simulink model "OLvsCL"  (Simulink 8.0)
settings: Solver=ode45  StartTime=0.0  StopTime=10.0  RelTol=1e-3
libraries: NbLibrary x10, cstblocks x7
settings Model: Creator=vaadya  LastModifiedBy=ccw
settings DataIOCC: SignalLoggingSaveFormat=ModelDataLogs
settings OptimizationCC: ExpressionDepthLimit=128
settings DebuggingCC: UnderspecifiedInitializationDetection=Simplified  MergeDetectMultiDrivingBlocksExec=error  SolverPrmCheckMsg=none  FcnCallInpInsideContextMsg=EnableAllAsWarning  FrameProcessingCompatibilityMsg=error  StateNameClashWarn=none
settings CodeAppCC: CustomSymbolStrType=$N$R$M_T
settings GRTTargetCC: CodeReplacementLibrary=C89/C90 (ANSI)  CombineOutputUpdateFcns=off  GRTInterface=on

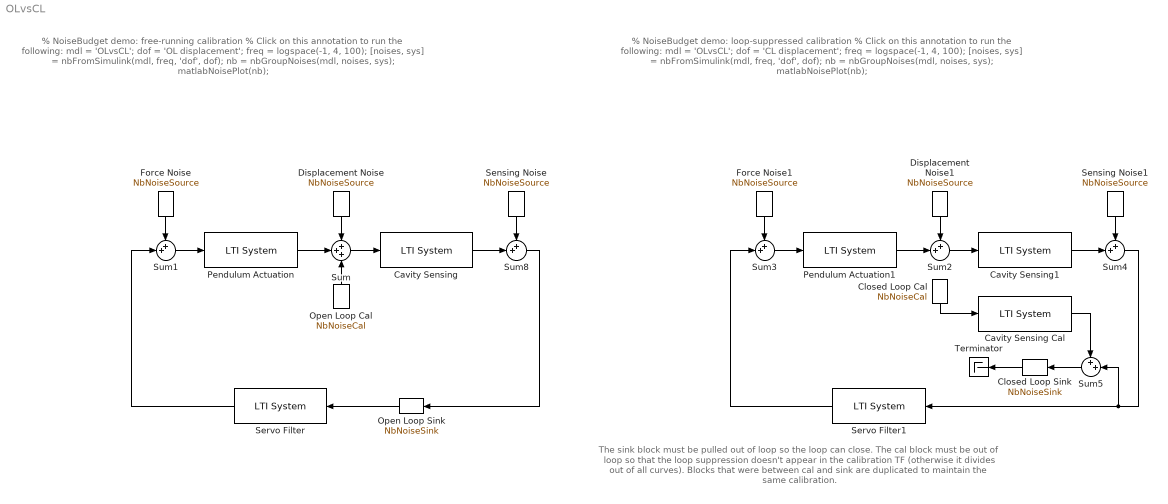
== system OLvsCL ==
  note: The sink block must be pulled out of loop so the loop can close.
      |
      | The cal block must be out of loop so that the loop suppression
      | doesn't appear in the calibration TF (otherwise it divides out of all
      | curves). Blocks that were between cal and sink are duplicated to
      | maintain the same calibration.
  note: % NoiseBudget demo: free-running calibration
      |   % Click on this annotation to run the following:
      |   mdl = 'OLvsCL';
      |   dof = 'OL displacement';
      |   freq = logspace(-1, 4, 100);
      |   [noises, sys] = nbFromSimulink(mdl, freq, 'dof', dof);
      |   nb = nbGroupNoises(mdl, noises, sys);
      |   matlabNoisePlot(nb);
  note: % NoiseBudget demo: loop-suppressed calibration
      |   % Click on this annotation to run the following:
      |   mdl = 'OLvsCL';
      |   dof = 'CL displacement';
      |   freq = logspace(-1, 4, 100);
      |   [noises, sys] = nbFromSimulink(mdl, freq, 'dof', dof);
      |   nb = nbGroupNoises(mdl, noises, sys);
      |   matlabNoisePlot(nb);
  Cavity Sensing : cstblocks/LTI System  sys=zpk([],-2*pi*[1000],2*pi*1000)  IC=[]
  Cavity Sensing Cal : cstblocks/LTI System  sys=zpk([],-2*pi*[1000],2*pi*1000)  IC=[]
  Cavity Sensing1 : cstblocks/LTI System  sys=zpk([],-2*pi*[1000],2*pi*1000)  IC=[]
  Closed Loop Cal : NbLibrary/NbNoiseCal  Tag=NbNoiseCal  dof='CL displacement'  unit='m/rtHz'
      settings: AttributesFormatString=%<Tag>
  Closed Loop Sink : NbLibrary/NbNoiseSink  Tag=NbNoiseSink  dof='CL displacement'  asd=''  chan=''
      settings: AttributesFormatString=%<Tag>
  Displacement Noise : NbLibrary/NbNoiseSource  Tag=NbNoiseSource  asd=2e-18  chan=''  groupNest=1  group=''  subgroup=''  subsubgroup=''  subsubsubgroup=''
      settings: AttributesFormatString=%<Tag>
  Displacement Noise1 : NbLibrary/NbNoiseSource  Tag=NbNoiseSource  asd=2e-18  chan=''  groupNest=1  group=''  subgroup=''  subsubgroup=''  subsubsubgroup=''
      settings: AttributesFormatString=%<Tag>
  Force Noise : NbLibrary/NbNoiseSource  Tag=NbNoiseSource  asd=1e-15  chan=''  groupNest=1  group=''  subgroup=''  subsubgroup=''  subsubsubgroup=''
      settings: AttributesFormatString=%<Tag>
  Force Noise1 : NbLibrary/NbNoiseSource  Tag=NbNoiseSource  asd=1e-15  chan=''  groupNest=1  group=''  subgroup=''  subsubgroup=''  subsubsubgroup=''
      settings: AttributesFormatString=%<Tag>
  Open Loop Cal : NbLibrary/NbNoiseCal  Tag=NbNoiseCal  dof='OL displacement'  unit='m/rtHz'
      settings: AttributesFormatString=%<Tag>
  Open Loop Sink : NbLibrary/NbNoiseSink  Tag=NbNoiseSink  dof='OL displacement'  asd=''  chan=''
      settings: AttributesFormatString=%<Tag>
  Pendulum Actuation : cstblocks/LTI System  sys=zpk([],-2*pi*[1 1],(2*pi)^2)  IC=[]
  Pendulum Actuation1 : cstblocks/LTI System  sys=zpk([],-2*pi*[1 1],(2*pi)^2)  IC=[]
  Sensing Noise : NbLibrary/NbNoiseSource  Tag=NbNoiseSource  asd=1e-18  chan=''  groupNest=1  group=''  subgroup=''  subsubgroup=''  subsubsubgroup=''
      settings: AttributesFormatString=%<Tag>
  Sensing Noise1 : NbLibrary/NbNoiseSource  Tag=NbNoiseSource  asd=1e-18  chan=''  groupNest=1  group=''  subgroup=''  subsubgroup=''  subsubsubgroup=''
      settings: AttributesFormatString=%<Tag>
  Servo Filter : cstblocks/LTI System  sys=zpk(-2*pi*[1],-2*pi*[1000],-1000*100)  IC=[]
  Servo Filter1 : cstblocks/LTI System  sys=zpk(-2*pi*[1],-2*pi*[1000],-1000*100)  IC=[]
  Sum : Sum  Inputs=+++
  Sum{1..5,8} (6 alike) : Sum  Inputs=++|
  Terminator : Terminator
  wires:
  Cavity Sensing/1 -> Sum8/2
  Pendulum Actuation/1 -> Sum/2
  Displacement Noise/1 -> Sum/1
  Sensing Noise/1 -> Sum8/1
  Open Loop Sink/1 -> Servo Filter/1
  Sum8/1 -> Open Loop Sink/1
  Sum1/1 -> Pendulum Actuation/1
  Servo Filter/1 -> Sum1/2
  Force Noise/1 -> Sum1/1
  Sum/1 -> Cavity Sensing/1
  Open Loop Cal/1 -> Sum/3
  Cavity Sensing1/1 -> Sum4/2
  Pendulum Actuation1/1 -> Sum2/2
  Displacement Noise1/1 -> Sum2/1
  Sensing Noise1/1 -> Sum4/1
  Sum3/1 -> Pendulum Actuation1/1
  Servo Filter1/1 -> Sum3/2
  Force Noise1/1 -> Sum3/1
  Closed Loop Sink/1 -> Terminator/1
  Sum5/1 -> Closed Loop Sink/1
  Cavity Sensing Cal/1 -> Sum5/1
  Sum4/1 -> Servo Filter1/1, Sum5/2
  Sum2/1 -> Cavity Sensing1/1
  Closed Loop Cal/1 -> Cavity Sensing Cal/1
